simulink model "PV_MPPT_BuckBoost"  (R2025b)
settings: Solver=VariableStepAuto  StartTime=0.0  StopTime=80  FixedStep=0.01  MaxStep=1e-3  MinStep=1e-13  RelTol=1e-2
libraries: AvgModels x3, slpidlib x1, simulink x1

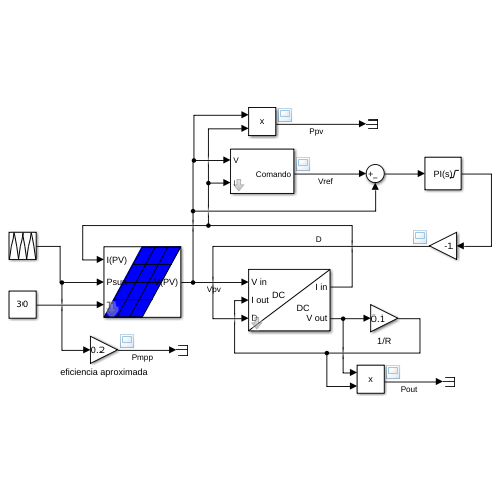
[thumbnail: Simulink's stored preview of the top-level diagram]
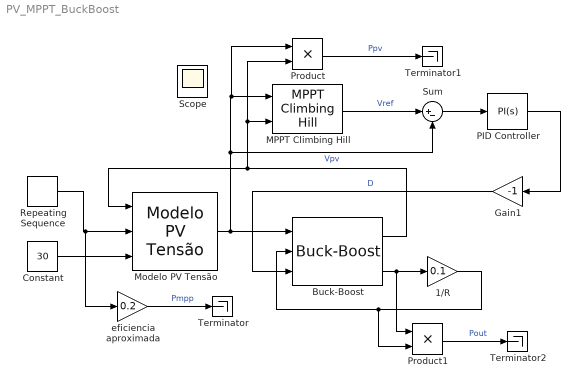
== system PV_MPPT_BuckBoost ==
  1/R : Gain  Gain=0.1
  Buck-Boost : AvgModels/Conversores Eletrônicos de Potência/Buck-Boost  C=1e-3  L=1e-4  RL=0.1  Edit_carga=1000  Vini=0  Iini=0  Fs=20000  Rdson=0  Vson=0  Rdon=0  Vdon=0.8
      settings: SourceProductName=SimAverageModels
  Constant : Constant  Value=30
  Gain1 : Gain  Gain=-1
  MPPT Climbing Hill : AvgModels/MPPT/MPPT Climbing Hill  fb=500  Passo=-2  limsup=30  liminf=20  Inicial=25
      settings: SourceProductName=SimAverageModels
  Modelo PV Tensão : AvgModels/Fontes/Modelo PV Tensão  Ns=54  Voc=0.6093  Isc=8.21  Rs=0.005  Rp=7  Ms=1  Mp=1  Tr=273 + 25  a=3.18e-3  n=1.2  k=1.38e-23  q=1.60e-19  EG=1.1  tau=1e-2  Psun=1000  Animar=off
      settings: SourceProductName=SimAverageModels
  PID Controller : slpidlib/PID Controller  Controller=PI  Form=Parallel  TimeDomain=Continuous-time  UseExternalTs=off  SampleTime=-1  IntegratorMethod=Forward Euler  FilterMethod=Forward Euler  ControllerParametersSource=internal  P=1/200  I=1/20  UseKiTs=off  D=0  UseExternalDerivativeSource=off  N=100  UseFilter=on  TunerSelectOption=Transfer Function Based (PID Tuner App)  InitialConditionSource=internal  InitialConditionForIntegrator=0  InitialConditionForFilter=0  DifferentiatorICPrevScaledInput=0  ExternalReset=none  TrackingMode=off  Kt=1  LimitOutput=on  SatLimitsSource=internal  UpperSaturationLimit=0  LowerSaturationLimit=-0.8  LinearizeAsGain=on  AntiWindupMode=none  Kb=1  LimitIntegrator=off  UpperIntegratorSaturationLimit=inf  LowerIntegratorSaturationLimit=-inf  POutMin=[]  POutMax=[]  IOutMin=[]  IOutMax=[]  DOutMin=[]  DOutMax=[]  NOutMin=[]  NOutMax=[]  SumOutMin=[]  SumOutMax=[]  SaturationOutMin=[]  SaturationOutMax=[]  PParamMin=[]  PParamMax=[]  IParamMin=[]  IParamMax=[]  DParamMin=[]  DParamMax=[]  NParamMin=[]  NParamMax=[]  KbParamMin=[]  KbParamMax=[]  KtParamMin=[]  KtParamMax=[]  KbOutMin=[]  KbOutMax=[]  KtOutMin=[]  KtOutMax=[]  IntegratorOutMin=[]  IntegratorOutMax=[]  FilterOutMin=[]  FilterOutMax=[]  SumI1OutMin=[]  SumI1OutMax=[]  SumI2OutMin=[]  SumI2OutMax=[]  SumI3OutMin=[]  SumI3OutMax=[]  SumI4OutMin=[]  SumI4OutMax=[]  SumDOutMin=[]  SumDOutMax=[]  DifferentiatorOutMin=[]  DifferentiatorOutMax=[]  FilterDiffOutCoefMin=[]  FilterDiffOutCoefMax=[]  ReciprocalOutMin=[]  ReciprocalOutMax=[]  SumDenOutMin=[]  SumDenOutMax=[]  SumNumOutMin=[]  SumNumOutMax=[]  DivideOutMin=[]  DivideOutMax=[]  UdiffTsProdOutMin=[]  UdiffTsProdOutMax=[]  NTsProdOutMin=[]  NTsProdOutMax=[]  UintegralTsProdOutMin=[]  UintegralTsProdOutMax=[]  UngainTsProdOutMin=[]  UngainTsProdOutMax=[]  ClampingZeroOutDataTypeStr=Inherit: Inherit via back propagation  ClampingZeroOutMin=[]  ClampingZeroOutMax=[]  FilterDenConstantOutDataTypeStr=Inherit: Inherit via back propagation  FilterDenConstantOutMin=[]  FilterDenConstantOutMax=[]  PCopyOutDataTypeStr=Inherit: Inherit via back propagation  PCopyOutMin=[]  PCopyOutMax=[]  NCopyOutDataTypeStr=Inherit: Inherit via back propagation  NCopyOutMin=[]  NCopyOutMax=[]  IntegratorContinuousStateAttributes=''  IntegratorStateMustResolveToSignalObject=off  IntegratorRTWStateStorageClass=Auto  FilterContinuousStateAttributes=''  FilterStateMustResolveToSignalObject=off  FilterRTWStateStorageClass=Auto  ParallelPVariant=InternalParameters  IdealPVariant=Disabled  IVariant=InternalParameters  DVariant=Disabled  IntegratorVariant=Continuous  SatVariant=Enabled  AWVariant=Passthrough  PCopyVariant=Disabled  TRVariant=Disabled  FdbkBlocksVariant=Forward  IdealPFdbkVariant=Disabled  SatFdbkVariant=Disabled  DerivativeFilterVariant=Disabled  NVariant=Disabled  NCopyVariant=Disabled_SignalSpec  FilterICVariant=Disabled  IntegratorICVariant=InternalICs  ExternalResetVariant=Disabled  TRSumVariant=Passthrough  SumFdbkVariant=Disabled  SumVariant=Sum_PI  TsampFilterVariant=InternalTs  TsampNgainVariant=Passthrough  TsampIntegralVariant=Disabled_SignalSpec  ExternalSaturationOutDataTypeStr=Inherit: Same as second input  DerivativeSourceVariant=Disabled  PreIntVariant=InternalPreInt
  Product : Product
  Product1 : Product
  Repeating Sequence : simulink/Sources/Repeating Sequence  rep_seq_t=[0 2 4 5 6 8 10]*4  rep_seq_y=[1 5 7 9 8 5 1]*100
  Sum : Sum  Inputs=|+-
  Terminator : Terminator
  Terminator1 : Terminator
  Terminator2 : Terminator
  eficiencia aproximada : Gain  Gain=0.2
  Scope : Scope
      settings: ActiveDisplayYMinimum=-3.75  ActiveDisplayYMaximum=33.75
  wires:
  Modelo PV Tensão/1 -> Buck-Boost/1, Sum/2, Product/1, MPPT Climbing Hill/1  "Vpv"
  Buck-Boost/1 -> Product/2, MPPT Climbing Hill/2, Modelo PV Tensão/1
  Buck-Boost/2 -> Product1/1, 1/R/1
  1/R/1 -> Product1/2, Buck-Boost/2
  MPPT Climbing Hill/1 -> Sum/1  "Vref"
  Sum/1 -> PID Controller/1
  PID Controller/1 -> Gain1/1
  Constant/1 -> Modelo PV Tensão/3
  Repeating Sequence/1 -> eficiencia aproximada/1, Modelo PV Tensão/2
  Gain1/1 -> Buck-Boost/3  "D"
  eficiencia aproximada/1 -> Terminator/1  "Pmpp"
  Product/1 -> Terminator1/1  "Ppv"
  Product1/1 -> Terminator2/1  "Pout"
